simulink model "USV_Trajectory_Tracking_Control_Model"  (R2020b)
settings: Solver=ode4  StartTime=0.0  StopTime=400  FixedStep=0.01  RelTol=1e-3
libraries: simulink x15, sharedutil x6, aerolibutil x1
settings Model: Creator=cdsouza  LastModifiedBy=Admin
settings SolverCC: ZeroCrossAlgorithm=Adaptive
settings DataIOCC: ReturnWorkspaceOutputs=off
settings DebuggingCC: MaskedZcDiagnostic=none  IgnoredZcDiagnostic=none  ArithmeticOperatorsInVariantConditions=warning
settings SFSimCC: CustomCodeUndefinedFunction=UseInterfaceOnly

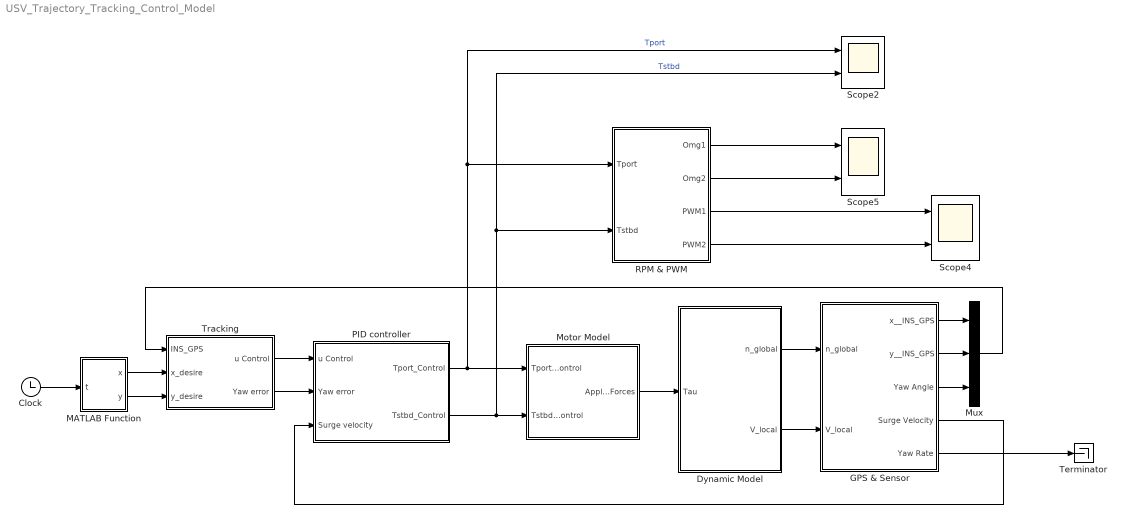
== system USV_Trajectory_Tracking_Control_Model ==
  Clock : Clock
  Dynamic Model : Subsystem
  GPS & Sensor : Subsystem
  MATLAB Function : MATLAB Function  TreatAsAtomicUnit=on
  Motor Model : Subsystem
  Mux : Mux  Inputs=3
  PID controller : Subsystem
  RPM & PWM : Subsystem
  Scope2 : Scope  NumInputPorts=2
  Scope4 : Scope  NumInputPorts=2
  Scope5 : Scope  NumInputPorts=2
  Terminator : Terminator
  Tracking : Subsystem
  wires:
  Tracking/1(u Control) -> PID controller/1(u Control)
  Tracking/2(Yaw error) -> PID controller/2(Yaw error)
  Dynamic Model/1(n_global) -> GPS & Sensor/1(n_global)
  Clock/1 -> MATLAB Function/1(t)
  MATLAB Function/1(x) -> Tracking/2(x_desire)
  MATLAB Function/2(y) -> Tracking/3(y_desire)
  PID controller/1(Tport_Control) -> Motor Model/1(Tport_Control), Scope2/1, RPM & PWM/1(Tport)  "Tport"
  PID controller/2(Tstbd_Control) -> Motor Model/2(Tstbd_Control), Scope2/2, RPM & PWM/2(Tstbd)  "Tstbd"
  GPS & Sensor/2(y__INS_GPS) -> Mux/2
  GPS & Sensor/1(x__INS_GPS) -> Mux/1
  GPS & Sensor/3(Yaw Angle) -> Mux/3
  Mux/1 -> Tracking/1(INS_GPS)
  GPS & Sensor/4(Surge Velocity) -> PID controller/3(Surge velocity)
  GPS & Sensor/5(Yaw Rate) -> Terminator/1
  RPM & PWM/3(PWM1) -> Scope4/1
  RPM & PWM/4(PWM2) -> Scope4/2
  Motor Model/1(Applied Forces) -> Dynamic Model/1(Tau)
  RPM & PWM/1(Omg1) -> Scope5/1
  RPM & PWM/2(Omg2) -> Scope5/2
  Dynamic Model/2(V_local) -> GPS & Sensor/2(V_local)

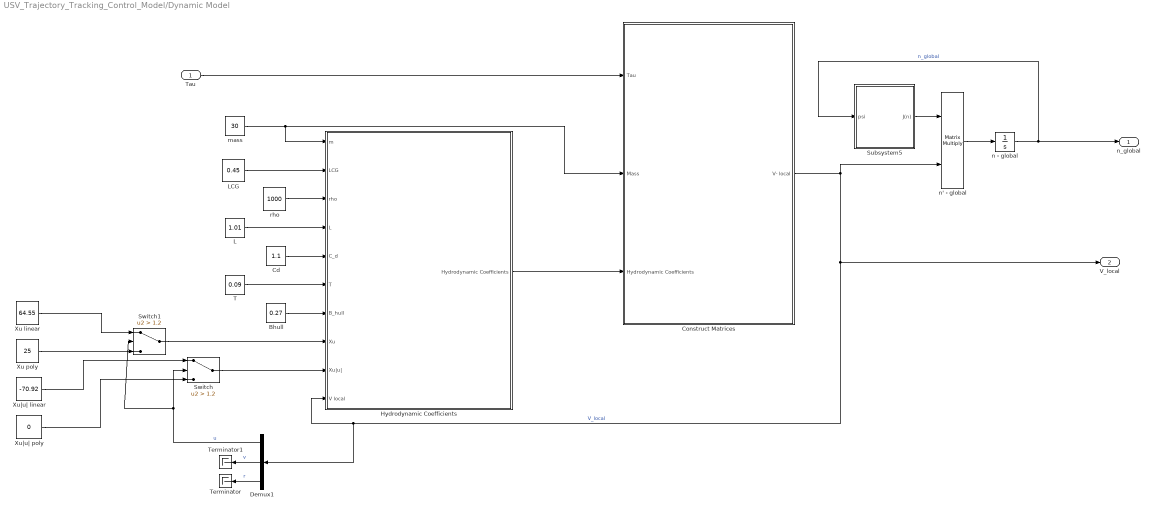
== system USV_Trajectory_Tracking_Control_Model/Dynamic Model ==
  Tau : Inport
  "Bhull " : Constant  Value=0.27
  Cd : Constant  Value=1.1
  Construct Matrices : Subsystem
  Demux1 : Demux  Outputs=3
  Hydrodynamic Coefficients : Subsystem
  L : Constant  Value=1.01
  LCG : Constant  Value=0.45
  Subsystem5 : Subsystem
  Switch : Switch  Criteria=u2 > Threshold  Threshold=1.2
  Switch1 : Switch  Criteria=u2 > Threshold  Threshold=1.2
  T : Constant  Value=0.09
  Terminator : Terminator
  Terminator1 : Terminator
  Xu linear : Constant  Value=64.55
  Xu poly : Constant  Value=25
  Xu|u| linear : Constant  Value=-70.92
  Xu|u| poly : Constant  Value=0
  mass : Constant  Value=30
  n - global : Integrator  InitialCondition=[0 0 0]
  n' - global : Product  Multiplication=Matrix(*)
  rho : Constant  Value=1000
  n_global : Outport  VectorParamsAs1DForOutWhenUnconnected=off
  V_local : Outport  Port=2  VectorParamsAs1DForOutWhenUnconnected=off
  wires:
  n - global/1 -> n_global/1, Subsystem5/1(psi)  "n_global"
  Cd/1 -> Hydrodynamic Coefficients/5(C_d)
  Construct Matrices/1(V- local) -> n' - global/2, Demux1/1, Hydrodynamic Coefficients/10(V local), V_local/1  "V_local"
  n' - global/1 -> n - global/1
  Subsystem5/1(J(n)) -> n' - global/1
  rho/1 -> Hydrodynamic Coefficients/3(rho)
  L/1 -> Hydrodynamic Coefficients/4(L)
  Tau/1 -> Construct Matrices/1(Tau)
  mass/1 -> Hydrodynamic Coefficients/1(m), Construct Matrices/2("Mass ")
  Hydrodynamic Coefficients/1("Hydrodynamic Coefficients ") -> Construct Matrices/3(Hydrodynamic Coefficients)
  T/1 -> Hydrodynamic Coefficients/6(T)
  "Bhull "/1 -> Hydrodynamic Coefficients/7(B_hull)
  Switch/1 -> Hydrodynamic Coefficients/9(Xu|u|)
  LCG/1 -> Hydrodynamic Coefficients/2(LCG)
  Demux1/1 -> Switch1/2, Switch/2  "u"
  Xu|u| poly/1 -> Switch/3
  Xu|u| linear/1 -> Switch/1
  Switch1/1 -> Hydrodynamic Coefficients/8(Xu)
  Xu poly/1 -> Switch1/3
  Xu linear/1 -> Switch1/1
  Demux1/3 -> Terminator/1  "r"
  Demux1/2 -> Terminator1/1  "v"

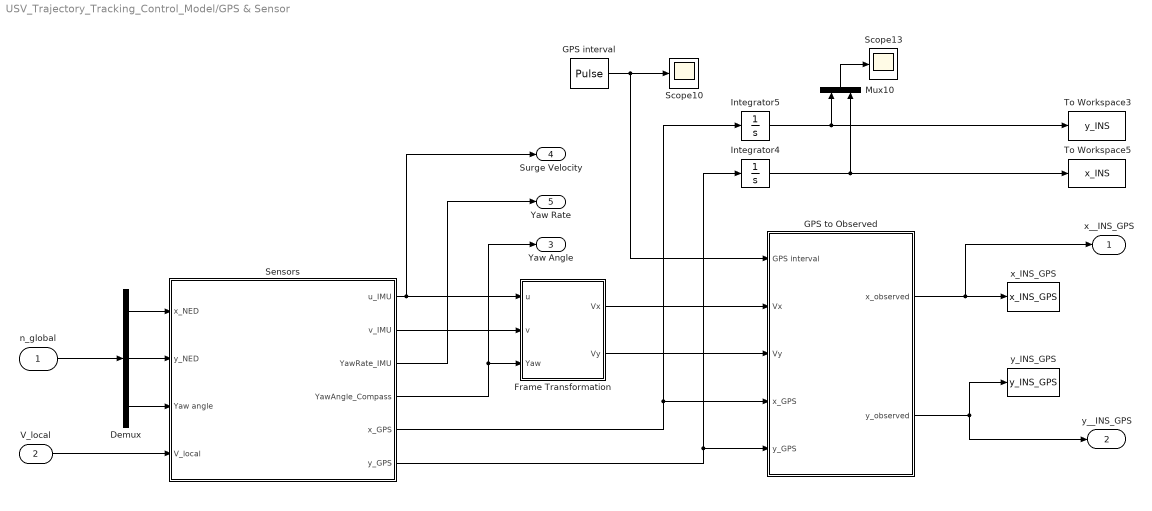
== system USV_Trajectory_Tracking_Control_Model/GPS & Sensor ==
  n_global : Inport
  V_local : Inport  Port=2
  Demux : Demux  Outputs=3
  Frame Transformation : Subsystem
  GPS interval : DiscretePulseGenerator  PulseType=Time based  Period=20  PulseWidth=5  PhaseDelay=0.2
  GPS to Observed : Subsystem
  Integrator4 : Integrator
  Integrator5 : Integrator
  Mux10 : Mux  Inputs=2
  Scope10 : Scope
  Scope13 : Scope
  Sensors : Subsystem
  To Workspace3 : ToWorkspace  VariableName=y_INS  SampleTime=-1
  To Workspace5 : ToWorkspace  VariableName=x_INS  SampleTime=-1
  x_INS_GPS : ToWorkspace  VariableName=x_INS_GPS  SampleTime=-1
  y_INS_GPS : ToWorkspace  VariableName=y_INS_GPS  SampleTime=-1
  x__INS_GPS : Outport  VectorParamsAs1DForOutWhenUnconnected=off
  y__INS_GPS : Outport  Port=2  VectorParamsAs1DForOutWhenUnconnected=off
  Yaw Angle : Outport  Port=3  VectorParamsAs1DForOutWhenUnconnected=off
  Surge Velocity : Outport  Port=4  VectorParamsAs1DForOutWhenUnconnected=off
  Yaw Rate : Outport  Port=5  VectorParamsAs1DForOutWhenUnconnected=off
  wires:
  GPS interval/1 -> GPS to Observed/1(GPS interval), Scope10/1
  Integrator5/1 -> To Workspace3/1, Mux10/1
  Sensors/1(u_IMU) -> Frame Transformation/1(u), Surge Velocity/1
  GPS to Observed/2(y_observed) -> y__INS_GPS/1, y_INS_GPS/1
  Mux10/1 -> Scope13/1
  GPS to Observed/1(x_observed) -> x__INS_GPS/1, x_INS_GPS/1
  Integrator4/1 -> To Workspace5/1, Mux10/2
  Sensors/2(v_IMU) -> Frame Transformation/2(v)
  Sensors/4(YawAngle_Compass) -> Yaw Angle/1, Frame Transformation/3(Yaw)
  Sensors/3(YawRate_IMU) -> Yaw Rate/1
  n_global/1 -> Demux/1
  Demux/3 -> Sensors/3(Yaw angle)
  Demux/1 -> Sensors/1(x_NED)
  Demux/2 -> Sensors/2(y_NED)
  V_local/1 -> Sensors/4(V_local)
  Sensors/6(y_GPS) -> Integrator4/1, GPS to Observed/5(y_GPS)
  Frame Transformation/2(Vy) -> GPS to Observed/3(Vy)
  Frame Transformation/1(Vx) -> GPS to Observed/2(Vx)
  Sensors/5(x_GPS) -> Integrator5/1, GPS to Observed/4(x_GPS)

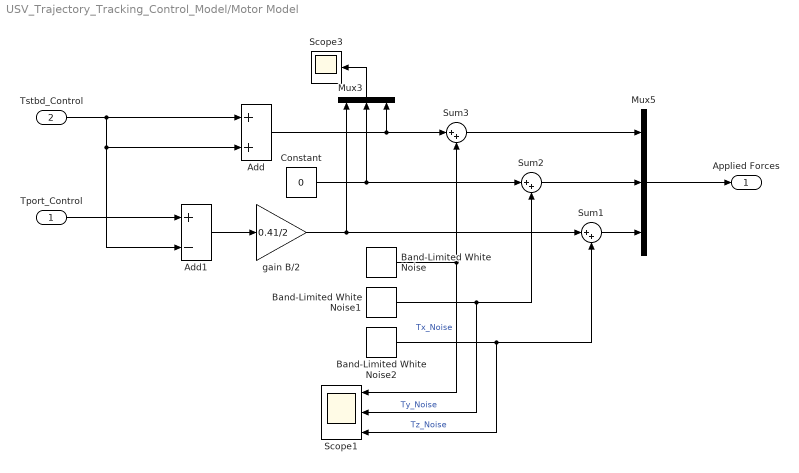
== system USV_Trajectory_Tracking_Control_Model/Motor Model ==
  Tport_Control : Inport
  Tstbd_Control : Inport  Port=2
  Add : Sum
  Add1 : Sum  Inputs=+-
  Band-Limited White Noise : simulink/Sources/Band-Limited White Noise  Cov=[0.05]  Ts=0.2  seed=[23341]
  Band-Limited White Noise1 : simulink/Sources/Band-Limited White Noise  Cov=[0.05]  Ts=0.2  seed=[23341]
  Band-Limited White Noise2 : simulink/Sources/Band-Limited White Noise  Cov=[0.05]  Ts=0.2  seed=[23341]
  Constant : Constant  Value=0
  Mux3 : Mux  Inputs=3
  Mux5 : Mux  Inputs=3
  Scope1 : Scope  NumInputPorts=3
  Scope3 : Scope
  Sum1 : Sum  Inputs=|++
  Sum2 : Sum  Inputs=|++
  Sum3 : Sum  Inputs=|++
  gain B/2 : Gain  Gain=0.41/2
  Applied Forces : Outport  VectorParamsAs1DForOutWhenUnconnected=off
  wires:
  Add1/1 -> gain B/2/1
  Tstbd_Control/1 -> Add1/2, Add/2, Add/1
  Add/1 -> Sum3/1, Mux3/3
  Tport_Control/1 -> Add1/1
  Constant/1 -> Mux3/2, Sum2/1
  Mux3/1 -> Scope3/1
  Band-Limited White Noise/1 -> Scope1/1, Sum3/2  "Tx_Noise"
  Mux5/1 -> Applied Forces/1
  Band-Limited White Noise2/1 -> Scope1/3, Sum1/2  "Tz_Noise"
  Sum3/1 -> Mux5/1
  Sum2/1 -> Mux5/2
  Sum1/1 -> Mux5/3
  gain B/2/1 -> Mux3/1, Sum1/1
  Band-Limited White Noise1/1 -> Scope1/2, Sum2/2  "Ty_Noise"

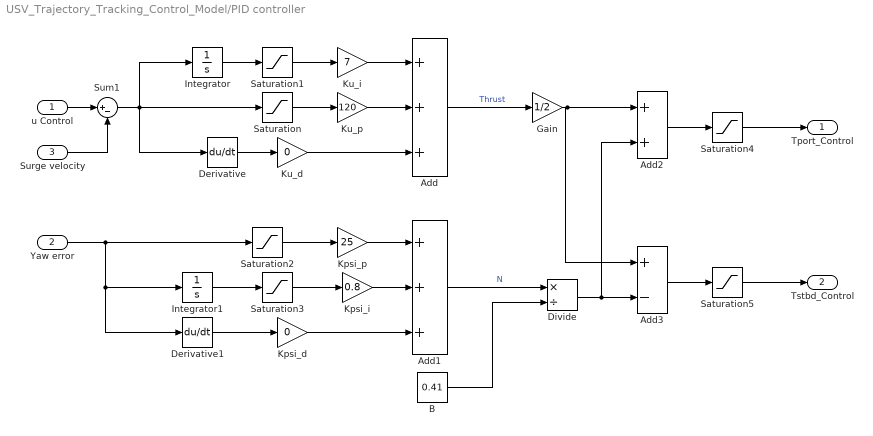
== system USV_Trajectory_Tracking_Control_Model/PID controller ==
  u Control : Inport
  Yaw error : Inport  Port=2
  Surge velocity : Inport  Port=3
  Add : Sum  Inputs=+++
  Add1 : Sum  Inputs=+++
  Add2 : Sum
  Add3 : Sum  Inputs=+-
  B : Constant  Value=0.41
  Derivative : Derivative
  Derivative1 : Derivative
  Divide : Product  Inputs=*/
  Gain : Gain  Gain=1/2
  Integrator : Integrator
  Integrator1 : Integrator
  Kpsi_d : Gain  Gain=0
  Kpsi_i : Gain  Gain=0.8
  Kpsi_p : Gain  Gain=25
  Ku_d : Gain  Gain=0
  Ku_i : Gain  Gain=7
  Ku_p : Gain  Gain=120
  Saturation : Saturate  UpperLimit=3  LowerLimit=0
  Saturation1 : Saturate  UpperLimit=10  LowerLimit=-10
  Saturation2 : Saturate  UpperLimit=0.8
  Saturation3 : Saturate  UpperLimit=10  LowerLimit=-10
  Saturation4 : Saturate  UpperLimit=25  LowerLimit=0
  Saturation5 : Saturate  UpperLimit=25  LowerLimit=0
  Sum1 : Sum  Inputs=|+-
  Tport_Control : Outport  VectorParamsAs1DForOutWhenUnconnected=off
  Tstbd_Control : Outport  Port=2  VectorParamsAs1DForOutWhenUnconnected=off
  wires:
  Integrator1/1 -> Saturation3/1
  Yaw error/1 -> Saturation2/1, Derivative1/1, Integrator1/1
  Surge velocity/1 -> Sum1/2
  u Control/1 -> Sum1/1
  Sum1/1 -> Derivative/1, Saturation/1, Integrator/1
  Integrator/1 -> Saturation1/1
  Saturation1/1 -> Ku_i/1
  Saturation/1 -> Ku_p/1
  Ku_p/1 -> Add/2
  Ku_i/1 -> Add/1
  Saturation2/1 -> Kpsi_p/1
  Saturation3/1 -> Kpsi_i/1
  Kpsi_p/1 -> Add1/1
  Kpsi_i/1 -> Add1/2
  Add/1 -> Gain/1  "Thrust"
  Add1/1 -> Divide/1  "N"
  B/1 -> Divide/2
  Gain/1 -> Add3/1, Add2/1
  Divide/1 -> Add3/2, Add2/2
  Add2/1 -> Saturation4/1
  Add3/1 -> Saturation5/1
  Derivative/1 -> Ku_d/1
  Ku_d/1 -> Add/3
  Derivative1/1 -> Kpsi_d/1
  Kpsi_d/1 -> Add1/3
  Saturation4/1 -> Tport_Control/1
  Saturation5/1 -> Tstbd_Control/1

== system USV_Trajectory_Tracking_Control_Model/RPM & PWM ==
  Tport : Inport
  Tstbd : Inport  Port=2
  Add : Sum
  Clock : Clock
  Constant : Constant  Value=3977
  Demux1 : Demux  Outputs=2
  Demux2 : Demux  Outputs=2
  Gain : Gain  Gain=1/(2e-6)
  Gain1 : Gain  Gain=1/79540
  Mux1 : Mux  Inputs=2
  PWM sim1 : MATLAB Function  TreatAsAtomicUnit=on
  PWM sim2 : MATLAB Function  TreatAsAtomicUnit=on
  Signed Square Root : Sqrt  Operator=signedSqrt  SaturateOnIntegerOverflow=on
  Omg1 : Outport
  Omg2 : Outport  Port=2
  PWM1 : Outport  Port=3
  PWM2 : Outport  Port=4
  wires:
  Mux1/1 -> Gain/1
  Tstbd/1 -> Mux1/2  "Tstbd"
  Tport/1 -> Mux1/1  "Tport"
  Gain/1 -> Signed Square Root/1
  Signed Square Root/1 -> Add/1, Demux2/1
  Add/1 -> Gain1/1
  Gain1/1 -> Demux1/1
  Demux1/1 -> PWM sim1/2(sig)
  Demux1/2 -> PWM sim2/2(sig)
  Clock/1 -> PWM sim2/1(rtime), PWM sim1/1(rtime)
  PWM sim1/1(pwm_wave) -> PWM1/1  "pwm"
  PWM sim2/1(pwm_wave) -> PWM2/1  "pwm"
  Constant/1 -> Add/2
  Demux2/1 -> Omg1/1
  Demux2/2 -> Omg2/1

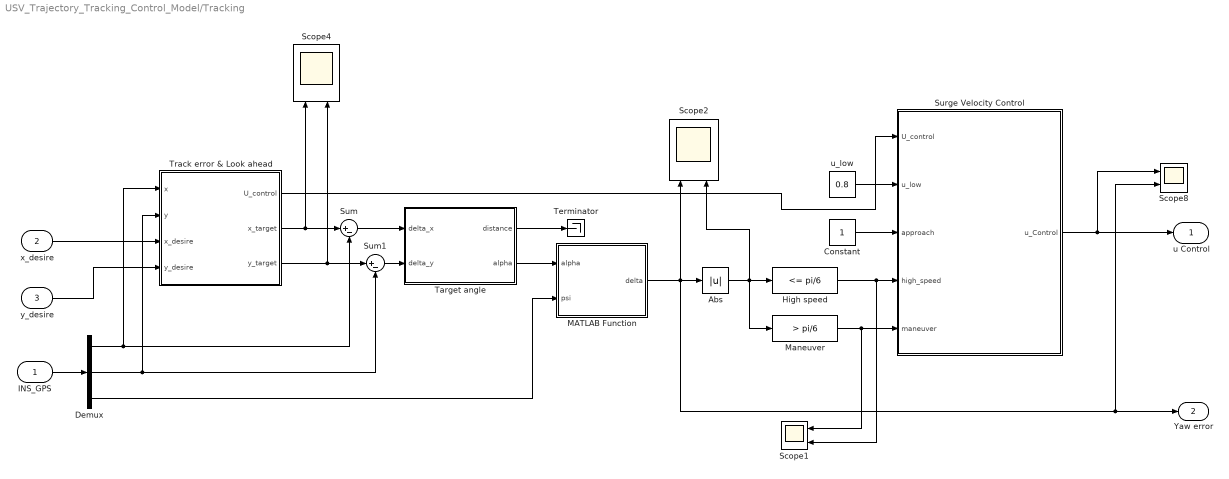
== system USV_Trajectory_Tracking_Control_Model/Tracking ==
  INS_GPS : Inport
  x_desire : Inport  Port=2
  y_desire : Inport  Port=3
  Abs : Abs
  Constant : Constant
  Demux : Demux  Outputs=3
  High speed : simulink/Logic and Bit Operations/Compare To Constant  relop=<=  const=pi/6  OutDataTypeStr=boolean
  MATLAB Function : MATLAB Function  TreatAsAtomicUnit=on
  Maneuver : simulink/Logic and Bit Operations/Compare To Constant  relop=>  const=pi/6  OutDataTypeStr=boolean
  Scope{1..2,4,8} (4 alike) : Scope  NumInputPorts=2
  Sum : Sum  Inputs=|+-
  Sum1 : Sum  Inputs=|+-
  Surge Velocity Control : MATLAB Function  TreatAsAtomicUnit=on
  Target angle : MATLAB Function  TreatAsAtomicUnit=on
  Terminator : Terminator
  Track error & Look ahead : Subsystem
  u_low : Constant  Value=0.8
  u Control : Outport  VectorParamsAs1DForOutWhenUnconnected=off
  Yaw error : Outport  Port=2  VectorParamsAs1DForOutWhenUnconnected=off
  wires:
  Target angle/2(alpha) -> MATLAB Function/1(alpha)
  Maneuver/1 -> Scope1/1, Surge Velocity Control/5(maneuver)
  Sum/1 -> Target angle/1(delta_x)
  u_low/1 -> Surge Velocity Control/2(u_low)
  Abs/1 -> High speed/1, Maneuver/1, Scope2/2
  Sum1/1 -> Target angle/2(delta_y)
  Demux/2 -> Sum1/2, Track error & Look ahead/2(y)
  MATLAB Function/1(delta) -> Scope2/1, Abs/1, Scope8/2, Yaw error/1
  High speed/1 -> Scope1/2, Surge Velocity Control/4(high_speed)
  Demux/1 -> Sum/2, Track error & Look ahead/1(x)
  Surge Velocity Control/1(u_Control) -> Scope8/1, u Control/1
  Demux/3 -> MATLAB Function/2(psi)
  Track error & Look ahead/2(x_target) -> Sum/1, Scope4/1
  Track error & Look ahead/3(y_target) -> Scope4/2, Sum1/1
  Target angle/1(distance) -> Terminator/1
  Track error & Look ahead/1(U_control) -> Surge Velocity Control/1(U_control)
  Constant/1 -> Surge Velocity Control/3(approach)
  INS_GPS/1 -> Demux/1
  x_desire/1 -> Track error & Look ahead/3(x_desire)
  y_desire/1 -> Track error & Look ahead/4(y_desire)

== system USV_Trajectory_Tracking_Control_Model/Dynamic Model/Construct Matrices ==
  note: v' local
  Tau : Inport
  "Mass " : Inport  Port=2
  Hydrodynamic Coefficients : Inport  Port=3
  I : Constant  Value=4.1
  Integrator : Integrator
  M : Subsystem
  M^-1 : aerolibutil/Invert  3x3 Matrix
  M^-1(T-C(v)-D(v)) : Product  Multiplication=Matrix(*)
  T-C(v)-D(v) : Subsystem
  XG : Constant  Value=0
  YG : Constant  Value=0
  V- local : Outport  VectorParamsAs1DForOutWhenUnconnected=off
  wires:
  M/1(M) -> M^-1/1  "M"
  Integrator/1 -> V- local/1, T-C(v)-D(v)/4(V_Local)  "V_Local"
  M^-1(T-C(v)-D(v))/1 -> Integrator/1
  I/1 -> M/4(I_z)
  M^-1/1 -> M^-1(T-C(v)-D(v))/1
  Hydrodynamic Coefficients/1 -> T-C(v)-D(v)/5(HydrodynamicCoefficients), M/5(Hydrodynamic coefficients)  "HydrodynamicCoefficients"
  YG/1 -> T-C(v)-D(v)/3(Y_G), M/3(Y_G)
  "Mass "/1 -> T-C(v)-D(v)/1(m), M/1(m)
  XG/1 -> T-C(v)-D(v)/2(X_G), M/2(X_G)
  T-C(v)-D(v)/1(Out1) -> M^-1(T-C(v)-D(v))/2
  Tau/1 -> T-C(v)-D(v)/6(Tau)

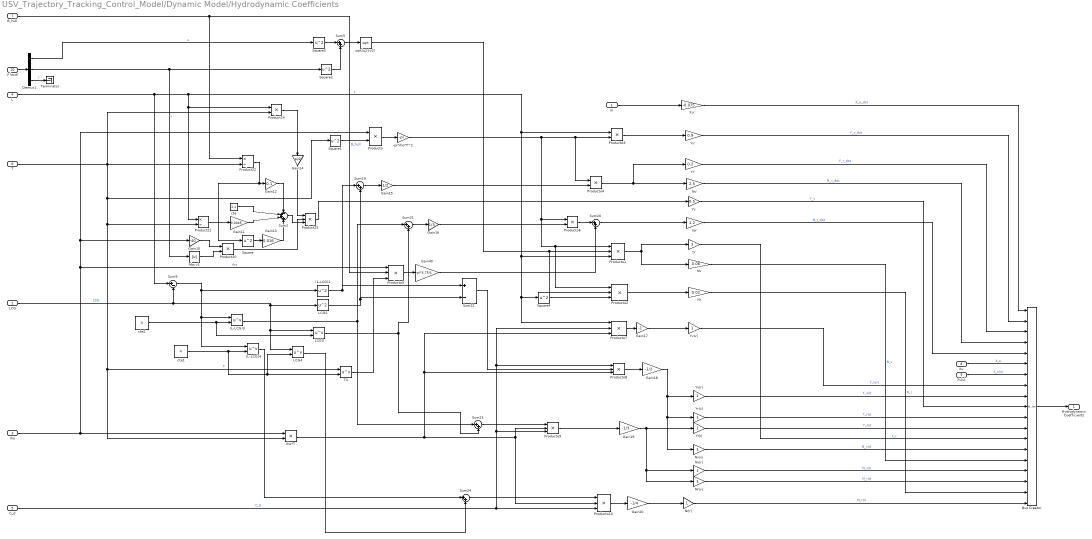
== system USV_Trajectory_Tracking_Control_Model/Dynamic Model/Hydrodynamic Coefficients ==
  m : Inport
  LCG : Inport  Port=2
  rho : Inport  Port=3
  L : Inport  Port=4
  C_d : Inport  Port=5
  T : Inport  Port=6
  B_hull : Inport  Port=7
  Xu : Inport  Port=8
  Xu|u| : Inport  Port=9
  V local : Inport  Port=10
  (L-LCG)2 : Math  Operator=square  SignedPower=on  SaturateOnIntegerOverflow=on
  (L-LCG)3 : Math  Operator=pow  SignedPower=on  SaturateOnIntegerOverflow=on
  (L-LCG)4 : Math  Operator=pow  SignedPower=on  SaturateOnIntegerOverflow=on
  -pi*rho*T^2 : Gain  Gain=-pi
  Abs v1 : Abs
  Bus Creator : BusCreator  Inputs=19
  Demux1 : Demux  Outputs=3
  Gain10 : Gain  Gain=-40
  Gain11 : Gain  Gain=0.0045
  Gain12 : Gain  Gain=0.1
  Gain13 : Gain  Gain=0.016
  Gain14 : Gain  Gain=pi/2
  Gain15 : Gain  Gain=1/2
  Gain16 : Gain  Gain=1/3
  Gain17 : Gain  Gain=-1
  Gain18 : Gain  Gain=-1/2
  Gain19 : Gain  Gain=-1/3
  Gain20 : Gain  Gain=-1/4
  Gain40 : Gain  Gain=-pi*4.75/4
  LCG2 : Math  Operator=square  SignedPower=on  SaturateOnIntegerOverflow=on
  LCG3 : Math  Operator=pow  SignedPower=on  SaturateOnIntegerOverflow=on
  LCG4 : Math  Operator=pow  SignedPower=on  SaturateOnIntegerOverflow=on
  Nr : Gain  Gain=0.02
  Nr' : Gain  Gain=1.2
  Nr|r| : Gain
  Nr|v| : Gain
  Nv : Gain  Gain=0.06
  Nv' : Gain  Gain=2.5
  Nv|r| : Gain
  Nv|v| : Gain
  Product20 : Product
  Product21 : Product  Inputs=*/
  Product22 : Product  Inputs=*/
  Product23 : Product  Inputs=3
  Product24 : Product
  Producto{,3..4,6} (4 alike) : Product
  Producto{1..2,5,7..10} (7 alike) : Product  Inputs=3
  Square{,1..4} (5 alike) : Math  Operator=square  SignedPower=on  SaturateOnIntegerOverflow=on
  Sum{5,19..21,23..24} (6 alike) : Sum  Inputs=|++
  Sum2 : Sum  Inputs=-+++
  Sum22 : Sum  Inputs=|+-
  Sum9 : Sum  Inputs=|+-
  T4 : Math  Operator=pow  SignedPower=on  SaturateOnIntegerOverflow=on
  Terminator : Terminator
  Xu' : Gain  Gain=-0.075
  Yr : Gain  Gain=3
  Yr' : Gain  Gain=0.2
  Yr|r| : Gain
  Yr|v| : Gain
  Yv : Gain  Gain=0.5
  Yv' : Gain  Gain=0.9
  Yv|r| : Gain
  Yv|v| : Gain
  cte : Constant  Value=1.1
  cte1 : Constant  Value=4
  cte2 : Constant  Value=3
  rho*T : Product
  sqrt(u2+v2) : Sqrt  SaturateOnIntegerOverflow=on
  "Hydrodynamic Coefficients " : Outport  VectorParamsAs1DForOutWhenUnconnected=off
  wires:
  m/1 -> Xu'/1
  Nv'/1 -> Bus Creator/4  "N_v_dot"
  Xu'/1 -> Bus Creator/1  "X_u_dot"
  Square/1 -> Gain13/1
  Gain14/1 -> Product23/1
  Product24/1 -> Gain14/1
  Sum9/1 -> (L-LCG)3/1, (L-LCG)4/1, (L-LCG)2/1
  Square4/1 -> Producto2/3
  sqrt(u2+v2)/1 -> Producto2/2, Producto1/2
  Product20/1 -> Product23/2
  Gain13/1 -> Sum2/4
  B_hull/1 -> Producto5/2, Product22/1  "B_hull"
  Square2/1 -> Sum5/2
  Sum20/1 -> Nr'/1
  Gain12/1 -> Sum2/1
  Sum21/1 -> Gain16/1
  LCG4/1 -> Sum24/2
  Sum24/1 -> Producto10/1
  (L-LCG)4/1 -> Sum24/1
  Sum2/1 -> Product23/3
  Producto10/1 -> Gain20/1
  (L-LCG)3/1 -> Sum21/1, Sum23/1
  Producto6/1 -> Sum20/1
  Gain19/1 -> Yr|r|/1, Nr|v|/1, Nv|r|/1
  Gain16/1 -> Producto6/2
  Sum22/1 -> Producto8/2
  Producto3/1 -> Yv'/1
  Gain10/1 -> Product20/1
  cte1/1 -> LCG4/2, T4/2, (L-LCG)4/2
  cte2/1 -> (L-LCG)3/2, LCG3/2
  Product23/1 -> Yv/1
  cte/1 -> Sum2/2
  Producto8/1 -> Gain18/1
  Sum23/1 -> Producto9/1
  Gain20/1 -> Nr|r|/1
  Gain18/1 -> Nv|v|/1, Yr|v|/1, Yv|r|/1
  Yr'/1 -> Bus Creator/3  "Y_r_dot"
  Producto7/1 -> Gain17/1
  Producto9/1 -> Gain19/1
  Gain11/1 -> Sum2/3
  Square1/1 -> Producto/2
  Producto2/1 -> Nr/1
  LCG3/1 -> Sum21/2, Sum23/2
  T4/1 -> Producto5/3
  Gain40/1 -> Sum20/2
  Producto4/1 -> Yr'/1, Nv'/1
  Sum19/1 -> Gain15/1
  Square3/1 -> Sum5/1
  Sum5/1 -> sqrt(u2+v2)/1
  rho/1 -> Producto/1, Gain10/1, Producto5/1, rho*T/1  "rho"
  Abs v1/1 -> Product20/2
  Product21/1 -> Gain11/1
  Gain17/1 -> Yv|v|/1
  (L-LCG)2/1 -> Sum19/1, Sum22/1
  Producto1/1 -> Nv/1, Yr/1
  Product22/1 -> Square/1, Gain12/1
  LCG2/1 -> Sum19/2, Sum22/2
  LCG/1 -> Sum9/2, LCG2/1, LCG3/1, LCG4/1  "LCG"
  Producto/1 -> -pi*rho*T^2/1
  -pi*rho*T^2/1 -> Producto4/1, Producto3/2, Producto2/1, Producto1/1, Producto6/1
  Producto5/1 -> Gain40/1
  Gain15/1 -> Producto4/2
  rho*T/1 -> Producto9/2, Producto10/2, Producto7/3, Producto8/3
  T/1 -> Product21/2, rho*T/2, T4/1, Square1/1, Product22/2, Product24/2  "T"
  L/1 -> Producto7/1, Square4/1, Producto1/3, Producto3/1, Product21/1, Product24/1, Sum9/1  "L"
  C_d/1 -> Producto7/2, Producto8/1, Producto9/3, Producto10/3  "C_d"
  Nv/1 -> Bus Creator/15  "N_v"
  Yv|v|/1 -> Bus Creator/8  "Y_v|v|"
  Yr|r|/1 -> Bus Creator/12  "Y_r|r|"
  Yv/1 -> Bus Creator/10  "Y_v"
  Nv|v|/1 -> Bus Creator/14  "N_v|v|"
  Yr|v|/1 -> Bus Creator/11  "Y_r|v|"
  Nv|r|/1 -> Bus Creator/16  "N_v|r|"
  Yr/1 -> Bus Creator/13  "Y_r"
  Nr|r|/1 -> Bus Creator/19  "N_r|r|"
  Nr/1 -> Bus Creator/18  "N_r"
  Xu|u|/1 -> Bus Creator/7  "X_u|u|"
  Yv|r|/1 -> Bus Creator/9  "Y_v|r|"
  Nr|v|/1 -> Bus Creator/17  "N_r|v|"
  Xu/1 -> Bus Creator/6  "X_u"
  Bus Creator/1 -> "Hydrodynamic Coefficients "/1
  Nr'/1 -> Bus Creator/5  "N_r_dot"
  Yv'/1 -> Bus Creator/2  "Y_v_dot"
  Demux1/1 -> Square3/1  "u"
  V local/1 -> Demux1/1
  Demux1/2 -> Abs v1/1, Square2/1  "v"
  Demux1/3 -> Terminator/1  "r"

== system USV_Trajectory_Tracking_Control_Model/Dynamic Model/Subsystem5 ==
  psi : Inport
  " J(n)" : sharedutil/Create 3x3 Matrix  aMode=aMode
      settings: SourceProductBaseCode=AE,PW,MT,UV,VE,VP
  Constant1 : Constant
  Constant2 : Constant  Value=0
  Gain9 : Gain  Gain=-1
  Selector : Selector  InputPortWidth=3  IndexOptions=Index vector (dialog)  Indices=3  OutputSizes=1
  Trigonometric Function : Trigonometry
  Trigonometric Function1 : Trigonometry  Operator=cos
  J(n) : Outport  VectorParamsAs1DForOutWhenUnconnected=off
  wires:
  Gain9/1 -> " J(n)"/2
  Trigonometric Function1/1 -> " J(n)"/5, " J(n)"/1
  Trigonometric Function/1 -> " J(n)"/4, Gain9/1
  Constant1/1 -> " J(n)"/9
  psi/1 -> Selector/1
  " J(n)"/1 -> J(n)/1
  Constant2/1 -> " J(n)"/8, " J(n)"/7, " J(n)"/6, " J(n)"/3
  Selector/1 -> Trigonometric Function1/1, Trigonometric Function/1

== system USV_Trajectory_Tracking_Control_Model/GPS & Sensor/Frame Transformation ==
  u : Inport
  v : Inport  Port=2
  Yaw : Inport  Port=3
  MATLAB Function : MATLAB Function  TreatAsAtomicUnit=on
  Vx : Outport  VectorParamsAs1DForOutWhenUnconnected=off
  Vy : Outport  Port=2  VectorParamsAs1DForOutWhenUnconnected=off
  wires:
  Yaw/1 -> MATLAB Function/3(Yaw)
  MATLAB Function/2(Vy_0) -> Vy/1
  u/1 -> MATLAB Function/1(u)
  MATLAB Function/1(Vx_0) -> Vx/1
  v/1 -> MATLAB Function/2(v)

== system USV_Trajectory_Tracking_Control_Model/GPS & Sensor/GPS to Observed ==
  GPS interval : Inport
  Vx : Inport  Port=2
  Vy : Inport  Port=3
  x_GPS : Inport  Port=4
  y_GPS : Inport  Port=5
  Mux6 : Mux  Inputs=2
  Scope8 : Scope
  x_inferred : Integrator  ExternalReset=rising  InitialConditionSource=external
  y_inferred : Integrator  ExternalReset=rising  InitialConditionSource=external
  x_observed : Outport  VectorParamsAs1DForOutWhenUnconnected=off
  y_observed : Outport  Port=2  VectorParamsAs1DForOutWhenUnconnected=off
  wires:
  y_inferred/1 -> y_observed/1, Mux6/1
  Vy/1 -> y_inferred/1
  GPS interval/1 -> y_inferred/2, x_inferred/2
  Vx/1 -> x_inferred/1
  x_inferred/1 -> x_observed/1, Mux6/2
  Mux6/1 -> Scope8/1
  y_GPS/1 -> y_inferred/3
  x_GPS/1 -> x_inferred/3

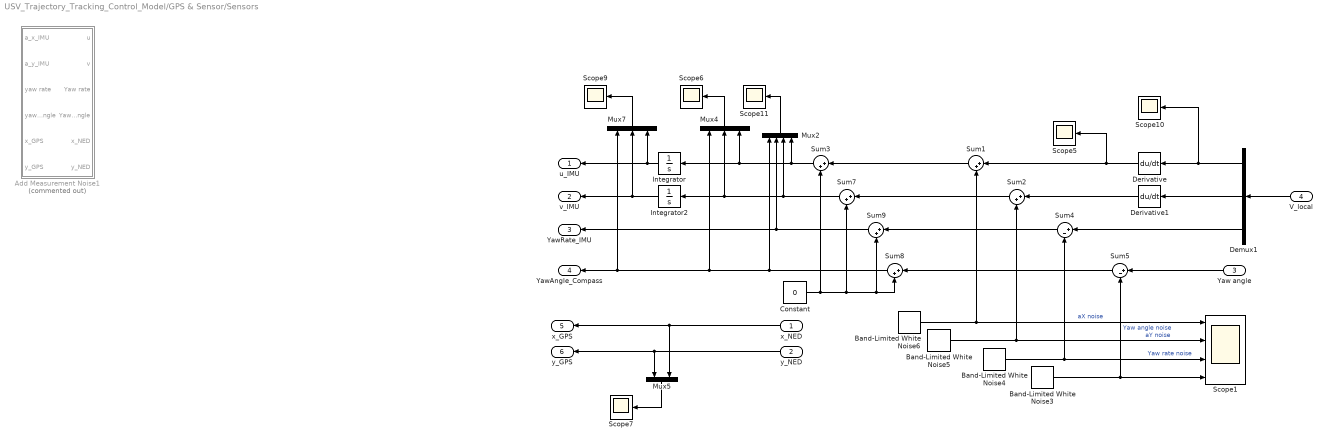
== system USV_Trajectory_Tracking_Control_Model/GPS & Sensor/Sensors ==
  x_NED : Inport
  y_NED : Inport  Port=2
  Yaw angle : Inport  Port=3
  V_local : Inport  Port=4
  Add Measurement Noise1 : Subsystem  Commented=on
  Band-Limited White Noise3 : simulink/Sources/Band-Limited White Noise  Cov=[0.0001]  Ts=0.1  seed=[23341]
  Band-Limited White Noise4 : simulink/Sources/Band-Limited White Noise  Cov=[0.00000001]  Ts=0.1  seed=[23341]
  Band-Limited White Noise5 : simulink/Sources/Band-Limited White Noise  Cov=[0.00000005]  Ts=0.1  seed=[23341]
  Band-Limited White Noise6 : simulink/Sources/Band-Limited White Noise  Cov=[0.000005]  Ts=0.1  seed=[23341]
  Constant : Constant  Value=0
  Demux1 : Demux  Outputs=3
  Derivative : Derivative
  Derivative1 : Derivative
  Integrator : Integrator
  Integrator2 : Integrator
  Mux2 : Mux
  Mux4 : Mux  Inputs=3
  Mux5 : Mux  Inputs=2
  Mux7 : Mux  Inputs=3
  Scope1 : Scope  NumInputPorts=4
  Scope{5..7,9..11} (6 alike) : Scope
  Sum{1..3,7..9} (6 alike) : Sum  Inputs=|++
  Sum4 : Sum  Inputs=|+-
  Sum5 : Sum  Inputs=|+-
  u_IMU : Outport  VectorParamsAs1DForOutWhenUnconnected=off
  v_IMU : Outport  Port=2  VectorParamsAs1DForOutWhenUnconnected=off
  YawRate_IMU : Outport  Port=3  VectorParamsAs1DForOutWhenUnconnected=off
  YawAngle_Compass : Outport  Port=4  VectorParamsAs1DForOutWhenUnconnected=off
  x_GPS : Outport  Port=5  VectorParamsAs1DForOutWhenUnconnected=off
  y_GPS : Outport  Port=6  VectorParamsAs1DForOutWhenUnconnected=off
  wires:
  Mux7/1 -> Scope9/1
  Sum3/1 -> Mux4/3, Integrator/1, Mux2/4
  Integrator/1 -> Mux7/3, u_IMU/1
  x_NED/1 -> Mux5/2, x_GPS/1
  Sum7/1 -> Mux4/2, Integrator2/1, Mux2/3
  Mux4/1 -> Scope6/1
  Integrator2/1 -> Mux7/2, v_IMU/1
  Mux5/1 -> Scope7/1
  Sum8/1 -> Mux2/1, Mux4/1, Mux7/1, YawAngle_Compass/1
  y_NED/1 -> y_GPS/1, Mux5/1
  Sum9/1 -> Mux2/2, YawRate_IMU/1
  V_local/1 -> Demux1/1
  Sum4/1 -> Sum9/1
  Sum5/1 -> Sum8/1
  Band-Limited White Noise6/1 -> Sum1/2, Scope1/1  "aX noise"
  Sum2/1 -> Sum7/1
  Mux2/1 -> Scope11/1
  Sum1/1 -> Sum3/1
  Band-Limited White Noise3/1 -> Sum5/2, Scope1/4  "Yaw angle noise"
  Demux1/3 -> Sum4/1
  Constant/1 -> Sum8/2, Sum9/2, Sum7/2, Sum3/2
  Derivative1/1 -> Sum2/1
  Demux1/1 -> Scope10/1, Derivative/1
  Yaw angle/1 -> Sum5/1
  Derivative/1 -> Scope5/1, Sum1/1
  Band-Limited White Noise5/1 -> Scope1/2, Sum2/2  "aY noise"
  Demux1/2 -> Derivative1/1
  Band-Limited White Noise4/1 -> Scope1/3, Sum4/2  "Yaw rate noise"

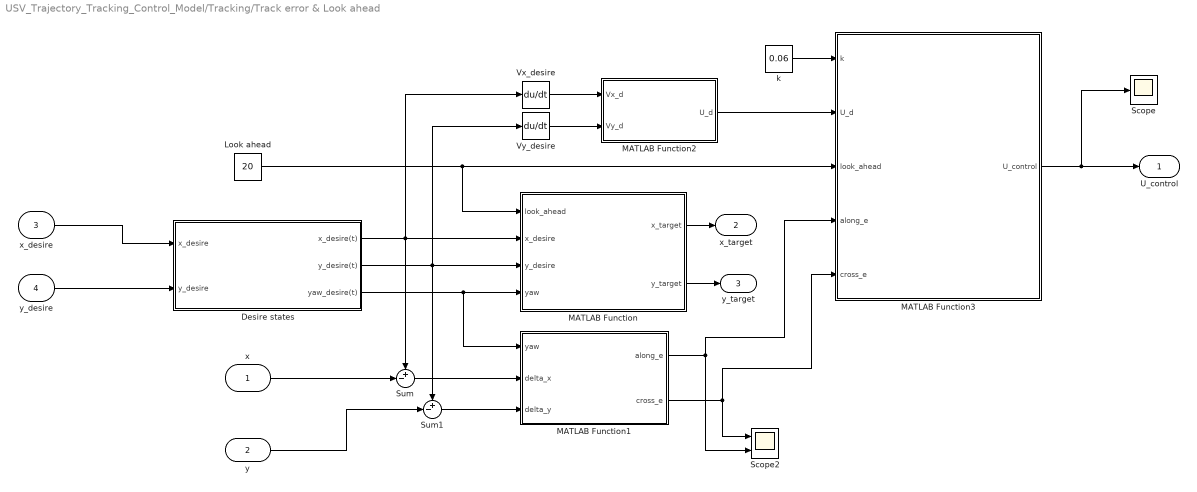
== system USV_Trajectory_Tracking_Control_Model/Tracking/Track error & Look ahead ==
  x : Inport
  y : Inport  Port=2
  x_desire : Inport  Port=3
  y_desire : Inport  Port=4
  Desire states : Subsystem
  Look ahead : Constant  Value=20
  MATLAB Function : MATLAB Function  TreatAsAtomicUnit=on
  MATLAB Function1 : MATLAB Function  TreatAsAtomicUnit=on
  MATLAB Function2 : MATLAB Function  TreatAsAtomicUnit=on
  MATLAB Function3 : MATLAB Function  TreatAsAtomicUnit=on
  Scope : Scope
  Scope2 : Scope  NumInputPorts=2
  Sum : Sum  Inputs=+-|
  Sum1 : Sum  Inputs=+-|
  Vx_desire : Derivative
  Vy_desire : Derivative
  k : Constant  Value=0.06
  U_control : Outport  VectorParamsAs1DForOutWhenUnconnected=off
  x_target : Outport  Port=2  VectorParamsAs1DForOutWhenUnconnected=off
  y_target : Outport  Port=3  VectorParamsAs1DForOutWhenUnconnected=off
  wires:
  Desire states/3(yaw_desire(t)) -> MATLAB Function1/1(yaw), MATLAB Function/4(yaw)
  Desire states/1(x_desire(t)) -> Vx_desire/1, MATLAB Function/2(x_desire), Sum/1
  Desire states/2(y_desire(t)) -> Sum1/1, MATLAB Function/3(y_desire), Vy_desire/1
  Look ahead/1 -> MATLAB Function/1(look_ahead), MATLAB Function3/3(look_ahead)
  MATLAB Function/1(x_target) -> x_target/1
  MATLAB Function/2(y_target) -> y_target/1
  x/1 -> Sum/2
  y/1 -> Sum1/2
  Sum1/1 -> MATLAB Function1/3(delta_y)
  Sum/1 -> MATLAB Function1/2(delta_x)
  Vx_desire/1 -> MATLAB Function2/1(Vx_d)
  Vy_desire/1 -> MATLAB Function2/2(Vy_d)
  MATLAB Function2/1(U_d) -> MATLAB Function3/2(U_d)
  MATLAB Function1/1(along_e) -> Scope2/2, MATLAB Function3/4(along_e)
  MATLAB Function1/2(cross_e) -> Scope2/1, MATLAB Function3/5(cross_e)
  k/1 -> MATLAB Function3/1(k)
  MATLAB Function3/1(U_control) -> Scope/1, U_control/1
  x_desire/1 -> Desire states/1(x_desire)
  y_desire/1 -> Desire states/2(y_desire)

== system USV_Trajectory_Tracking_Control_Model/Dynamic Model/Construct Matrices/M ==
  m : Inport
  X_G : Inport  Port=2
  Y_G : Inport  Port=3
  I_z : Inport  Port=4
  Hydrodynamic coefficients : Inport  Port=5
  Bus Selector : BusSelector  OutputSignals=X_u_dot,Y_r_dot,N_v_dot,Y_v_dot,N_r_dot
  Constant3 : Constant  Value=0
  Gain8 : Gain  Gain=-1
  Matrix M : sharedutil/Create 3x3 Matrix  aMode=aMode
      settings: SourceProductBaseCode=AE,PW,MT,UV,VE,VP
  Product17 : Product
  Product18 : Product
  Sum14 : Sum  Inputs=|+-
  Sum15 : Sum  Inputs=+-
  Sum16 : Sum  Inputs=+-
  Sum17 : Sum  Inputs=+-
  Sum18 : Sum  Inputs=|+-
  M : Outport  VectorParamsAs1DForOutWhenUnconnected=off
  wires:
  Gain8/1 -> Matrix M/7, Matrix M/3
  Product17/1 -> Gain8/1
  Product18/1 -> Sum17/1, Sum16/1
  Sum18/1 -> Matrix M/9
  Constant3/1 -> Matrix M/4, Matrix M/2
  I_z/1 -> Sum18/1  "I_z"
  Sum15/1 -> Matrix M/5
  m/1 -> Sum14/1, Product17/1, Sum15/1, Product18/1  "m"
  Bus Selector/3 -> Sum17/2  "<N_v_dot>"
  Sum14/1 -> Matrix M/1
  Sum16/1 -> Matrix M/6
  Matrix M/1 -> M/1
  Sum17/1 -> Matrix M/8
  X_G/1 -> Product18/2  "X_G"
  Y_G/1 -> Product17/2  "Y_G"
  Bus Selector/1 -> Sum14/2  "<X_u_dot>"
  Hydrodynamic coefficients/1 -> Bus Selector/1
  Bus Selector/2 -> Sum16/2  "<Y_r_dot>"
  Bus Selector/4 -> Sum15/2  "<Y_v_dot>"
  Bus Selector/5 -> Sum18/2  "<N_r_dot>"

== system USV_Trajectory_Tracking_Control_Model/Dynamic Model/Construct Matrices/T-C(v)-D(v) ==
  m : Inport
  X_G : Inport  Port=2
  Y_G : Inport  Port=3
  V_Local : Inport  Port=4
  HydrodynamicCoefficients : Inport  Port=5
  Tau : Inport  Port=6
  C : Subsystem
  C(v)v : Product  Multiplication=Matrix(*)
  D : Subsystem
  D(v)v : Product  Multiplication=Matrix(*)
  T - C(v)v - D(v)v : Sum  Inputs=+--
  Out1 : Outport  VectorParamsAs1DForOutWhenUnconnected=off
  wires:
  V_Local/1 -> D(v)v/2, C(v)v/2, D/2(V - local), C/5(V local)
  T - C(v)v - D(v)v/1 -> Out1/1
  D(v)v/1 -> T - C(v)v - D(v)v/3
  C(v)v/1 -> T - C(v)v - D(v)v/2
  C/1(C(v)) -> C(v)v/1  "C(v)"
  D/1(D(v)) -> D(v)v/1  "D(v)"
  HydrodynamicCoefficients/1 -> C/4(Hydrodynamic coefficients), D/1(Hydrodynamic Coefficients)
  Y_G/1 -> C/3(Y_G)
  X_G/1 -> C/2(X_G)
  m/1 -> C/1(m)
  Tau/1 -> T - C(v)v - D(v)v/1

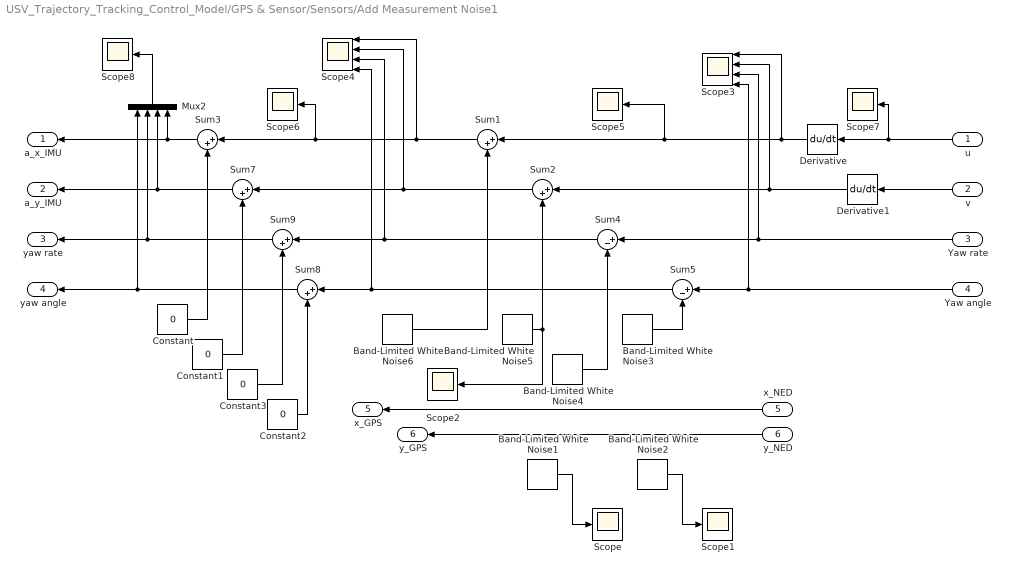
== system USV_Trajectory_Tracking_Control_Model/GPS & Sensor/Sensors/Add Measurement Noise1 ==
  u : Inport
  v : Inport  Port=2
  Yaw rate : Inport  Port=3
  Yaw angle : Inport  Port=4
  x_NED : Inport  Port=5
  y_NED : Inport  Port=6
  Band-Limited White Noise1 : simulink/Sources/Band-Limited White Noise  Cov=[0.5]  Ts=1  seed=[23341]
  Band-Limited White Noise2 : simulink/Sources/Band-Limited White Noise  Cov=[0.5]  Ts=1  seed=[23341]
  Band-Limited White Noise3 : simulink/Sources/Band-Limited White Noise  Cov=[0.0001]  Ts=0.1  seed=[23341]
  Band-Limited White Noise4 : simulink/Sources/Band-Limited White Noise  Cov=[0.00000001]  Ts=0.1  seed=[23341]
  Band-Limited White Noise5 : simulink/Sources/Band-Limited White Noise  Cov=[0.00000005]  Ts=0.1  seed=[23341]
  Band-Limited White Noise6 : simulink/Sources/Band-Limited White Noise  Cov=[0.000005]  Ts=0.1  seed=[23341]
  Constant{,1..3} (4 alike) : Constant  Value=0
  Derivative : Derivative
  Derivative1 : Derivative
  Mux2 : Mux
  Scope{,1..2,5..8} (7 alike) : Scope
  Scope3 : Scope  NumInputPorts=4
  Scope4 : Scope  NumInputPorts=4
  Sum{1..3,7..9} (6 alike) : Sum  Inputs=|++
  Sum4 : Sum  Inputs=|+-
  Sum5 : Sum  Inputs=|+-
  a_x_IMU : Outport  VectorParamsAs1DForOutWhenUnconnected=off
  a_y_IMU : Outport  Port=2  VectorParamsAs1DForOutWhenUnconnected=off
  yaw rate : Outport  Port=3  VectorParamsAs1DForOutWhenUnconnected=off
  yaw angle : Outport  Port=4  VectorParamsAs1DForOutWhenUnconnected=off
  x_GPS : Outport  Port=5  VectorParamsAs1DForOutWhenUnconnected=off
  y_GPS : Outport  Port=6  VectorParamsAs1DForOutWhenUnconnected=off
  wires:
  y_NED/1 -> y_GPS/1
  x_NED/1 -> x_GPS/1
  Band-Limited White Noise6/1 -> Sum1/2
  Sum2/1 -> Sum7/1, Scope4/2
  Sum4/1 -> Sum9/1, Scope4/3
  Band-Limited White Noise4/1 -> Sum4/2
  Sum5/1 -> Sum8/1, Scope4/4
  Band-Limited White Noise3/1 -> Sum5/2
  Sum1/1 -> Sum3/1, Scope6/1, Scope4/1
  Constant3/1 -> Sum9/2
  Sum9/1 -> yaw rate/1, Mux2/2
  Sum8/1 -> yaw angle/1, Mux2/1
  Yaw rate/1 -> Scope3/3, Sum4/1
  Sum7/1 -> a_y_IMU/1, Mux2/3
  Sum3/1 -> a_x_IMU/1, Mux2/4
  Mux2/1 -> Scope8/1
  Constant2/1 -> Sum8/2
  Constant1/1 -> Sum7/2
  Constant/1 -> Sum3/2
  Band-Limited White Noise2/1 -> Scope1/1
  Band-Limited White Noise1/1 -> Scope/1
  Derivative/1 -> Scope5/1, Sum1/1, Scope3/1
  Derivative1/1 -> Scope3/2, Sum2/1
  Yaw angle/1 -> Scope3/4, Sum5/1
  v/1 -> Derivative1/1
  u/1 -> Derivative/1, Scope7/1
  Band-Limited White Noise5/1 -> Sum2/2, Scope2/1

== system USV_Trajectory_Tracking_Control_Model/Tracking/Track error & Look ahead/Desire states ==
  x_desire : Inport
  y_desire : Inport  Port=2
  Derivative : Derivative
  Derivative1 : Derivative
  MATLAB Function : MATLAB Function  TreatAsAtomicUnit=on
  To Workspace : ToWorkspace  VariableName=x_desire  SampleTime=-1
  To Workspace1 : ToWorkspace  VariableName=y_desire  SampleTime=-1
  To Workspace2 : ToWorkspace  VariableName=yaw_desire  SampleTime=-1
  x_desire(t) : Outport  VectorParamsAs1DForOutWhenUnconnected=off
  y_desire(t) : Outport  Port=2  VectorParamsAs1DForOutWhenUnconnected=off
  yaw_desire(t) : Outport  Port=3  VectorParamsAs1DForOutWhenUnconnected=off
  wires:
  x_desire/1 -> Derivative/1, To Workspace/1, x_desire(t)/1
  y_desire/1 -> Derivative1/1, To Workspace1/1, y_desire(t)/1
  Derivative/1 -> MATLAB Function/1(dx)
  Derivative1/1 -> MATLAB Function/2(dy)
  MATLAB Function/1(yaw) -> To Workspace2/1, yaw_desire(t)/1

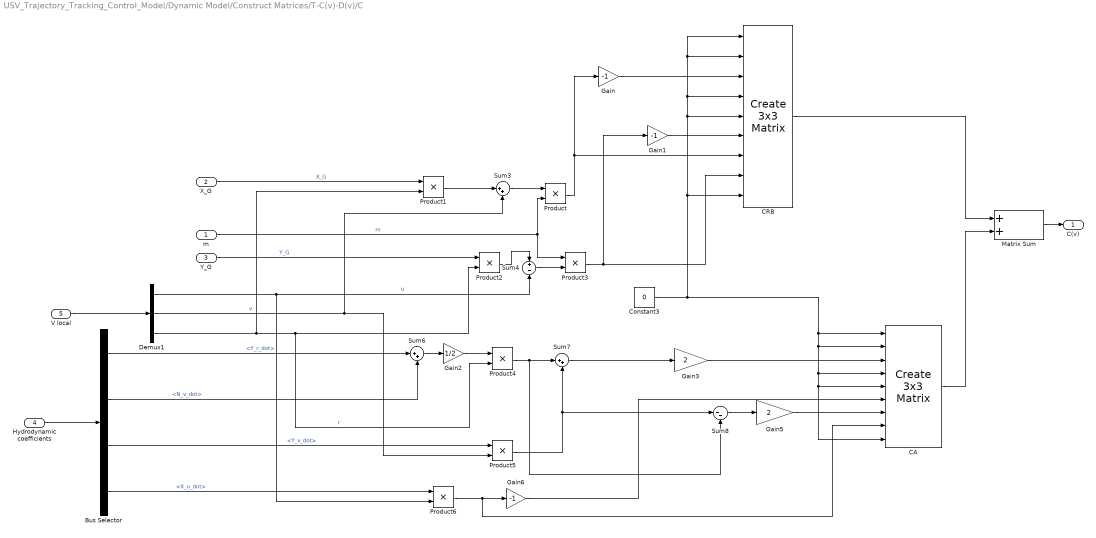
== system USV_Trajectory_Tracking_Control_Model/Dynamic Model/Construct Matrices/T-C(v)-D(v)/C ==
  m : Inport
  X_G : Inport  Port=2
  Y_G : Inport  Port=3
  Hydrodynamic coefficients : Inport  Port=4
  V local : Inport  Port=5
  " CRB" : sharedutil/Create 3x3 Matrix  aMode=aMode
      settings: SourceProductBaseCode=AE,PW,MT,UV,VE,VP
  Bus Selector : BusSelector  OutputSignals=Y_r_dot,N_v_dot,Y_v_dot,X_u_dot
  CA : sharedutil/Create 3x3 Matrix  aMode=aMode
      settings: SourceProductBaseCode=AE,PW,MT,UV,VE,VP
  Constant3 : Constant  Value=0
  Demux1 : Demux  Outputs=3
  Gain : Gain  Gain=-1
  Gain1 : Gain  Gain=-1
  Gain2 : Gain  Gain=1/2
  Gain3 : Gain  Gain=2
  Gain5 : Gain  Gain=2
  Gain6 : Gain  Gain=-1
  Matrix Sum : Sum
  Product{,1..6} (7 alike) : Product
  Sum3 : Sum  Inputs=|++
  Sum4 : Sum  Inputs=+-
  Sum6 : Sum  Inputs=|++
  Sum7 : Sum  Inputs=|++
  Sum8 : Sum  Inputs=|--
  C(v) : Outport  VectorParamsAs1DForOutWhenUnconnected=off
  wires:
  Bus Selector/1 -> Sum6/1  "<Y_r_dot>"
  Demux1/3 -> Product1/2, Product2/2, Product4/2  "r"
  Gain2/1 -> Product4/1
  CA/1 -> Matrix Sum/2
  Gain/1 -> " CRB"/3
  Bus Selector/2 -> Sum6/2  "<N_v_dot>"
  Sum3/1 -> Product/1
  Sum8/1 -> Gain5/1
  Product2/1 -> Sum4/1
  Sum6/1 -> Gain2/1
  Product5/1 -> Sum7/2, Sum8/1
  Gain1/1 -> " CRB"/6
  Product1/1 -> Sum3/1
  Y_G/1 -> Product2/1  "Y_G"
  Matrix Sum/1 -> C(v)/1
  Gain3/1 -> CA/3
  Gain6/1 -> CA/6
  Product6/1 -> Gain6/1, CA/8
  Demux1/2 -> Sum3/2, Product5/2  "v"
  Product4/1 -> Sum7/1, Sum8/2
  Product3/1 -> " CRB"/8, Gain1/1
  Gain5/1 -> CA/7
  " CRB"/1 -> Matrix Sum/1
  X_G/1 -> Product1/1  "X_G"
  Sum7/1 -> Gain3/1
  Product/1 -> " CRB"/7, Gain/1
  m/1 -> Product/2, Product3/1  "m"
  Constant3/1 -> " CRB"/5, " CRB"/4, " CRB"/2, " CRB"/1, " CRB"/9, CA/4, CA/5, CA/9, CA/2, CA/1
  Hydrodynamic coefficients/1 -> Bus Selector/1
  Bus Selector/4 -> Product6/1  "<X_u_dot>"
  Bus Selector/3 -> Product5/1  "<Y_v_dot>"
  Demux1/1 -> Sum4/2, Product6/2  "u"
  V local/1 -> Demux1/1
  Sum4/1 -> Product3/2

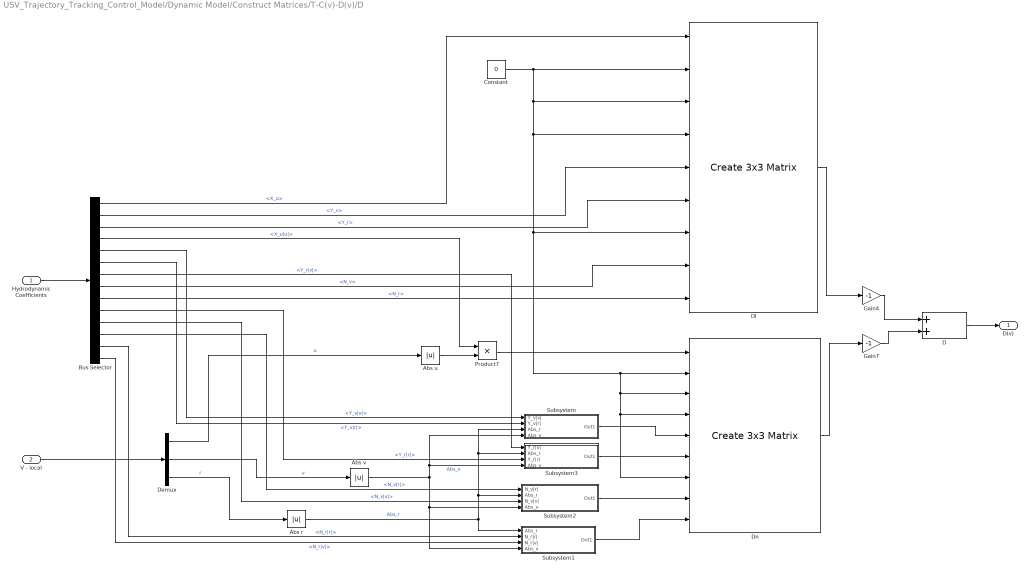
== system USV_Trajectory_Tracking_Control_Model/Dynamic Model/Construct Matrices/T-C(v)-D(v)/D ==
  Hydrodynamic Coefficients : Inport
  V - local : Inport  Port=2
  Abs r : Abs
  Abs u : Abs
  Abs v : Abs
  Bus Selector : BusSelector  OutputSignals=X_u,Y_v,Y_r,X_u|u|,Y_v|v|,Y_v|r|,Y_r|v|,N_v,N_r,Y_r|r|,N_v|v|,N_v|r|,N_r|r|,N_r|v|
  Constant : Constant  Value=0
  D : Sum
  Demux : Demux  Outputs=3
  Dl : sharedutil/Create 3x3 Matrix  aMode=aMode
      settings: SourceProductBaseCode=AE,PW,MT,UV,VE,VP
  Dn : sharedutil/Create 3x3 Matrix  aMode=aMode
      settings: SourceProductBaseCode=AE,PW,MT,UV,VE,VP
  Gain4 : Gain  Gain=-1
  Gain7 : Gain  Gain=-1
  Product7 : Product
  Subsystem : Subsystem
  Subsystem1 : Subsystem
  Subsystem2 : Subsystem
  Subsystem3 : Subsystem
  D(v) : Outport  VectorParamsAs1DForOutWhenUnconnected=off
  wires:
  Constant/1 -> Dn/7, Dn/4, Dn/3, Dn/2, Dl/7, Dl/4, Dl/3, Dl/2
  Abs u/1 -> Product7/2
  Abs r/1 -> Subsystem/3(Abs_r), Subsystem3/2("Abs_r "), Subsystem2/2(Abs_r), Subsystem1/1(Abs_r)  "Abs_r"
  Product7/1 -> Dn/1
  Abs v/1 -> Subsystem/4("Abs_v "), Subsystem3/4(Abs_v), Subsystem1/4(Abs_v), Subsystem2/4(Abs_v)  "Abs_v"
  Gain7/1 -> D/2
  Gain4/1 -> D/1
  Dl/1 -> Gain4/1
  Dn/1 -> Gain7/1
  D/1 -> D(v)/1
  Subsystem/1(Out1) -> Dn/5
  Subsystem1/1(Out1) -> Dn/9
  Subsystem2/1(Out1) -> Dn/8
  Subsystem3/1(Out1) -> Dn/6
  Hydrodynamic Coefficients/1 -> Bus Selector/1
  Bus Selector/5 -> Subsystem/1("Y_v|v| ")  "<Y_v|v|>"
  Bus Selector/6 -> Subsystem/2(Y_v|r|)  "<Y_v|r|>"
  Bus Selector/2 -> Dl/5  "<Y_v>"
  Bus Selector/7 -> Subsystem3/1(Y_r|v|)  "<Y_r|v|>"
  Bus Selector/10 -> Subsystem3/3(Y_r|r|)  "<Y_r|r|>"
  Bus Selector/11 -> Subsystem2/3(N_v|v|)  "<N_v|v|>"
  Bus Selector/8 -> Dl/8  "<N_v>"
  Bus Selector/12 -> Subsystem2/1(N_v|r|)  "<N_v|r|>"
  Bus Selector/14 -> Subsystem1/3(N_r|v|)  "<N_r|v|>"
  Bus Selector/9 -> Dl/9  "<N_r>"
  Bus Selector/13 -> Subsystem1/2(N_r|r|)  "<N_r|r|>"
  Bus Selector/1 -> Dl/1  "<X_u>"
  Bus Selector/4 -> Product7/1  "<X_u|u|>"
  Bus Selector/3 -> Dl/6  "<Y_r>"
  Demux/1 -> Abs u/1  "u"
  Demux/2 -> Abs v/1  "v"
  Demux/3 -> Abs r/1  "r"
  V - local/1 -> Demux/1

== system USV_Trajectory_Tracking_Control_Model/Dynamic Model/Construct Matrices/T-C(v)-D(v)/D/Subsystem ==
  "Y_v|v| " : Inport
  Y_v|r| : Inport  Port=2
  Abs_r : Inport  Port=3
  "Abs_v " : Inport  Port=4
  Product8 : Product
  Product9 : Product
  Sum10 : Sum  Inputs=|++
  Out1 : Outport  VectorParamsAs1DForOutWhenUnconnected=off
  wires:
  Y_v|r|/1 -> Product9/1
  Abs_r/1 -> Product9/2
  Product9/1 -> Sum10/2
  "Y_v|v| "/1 -> Product8/1
  Product8/1 -> Sum10/1
  "Abs_v "/1 -> Product8/2
  Sum10/1 -> Out1/1

== system USV_Trajectory_Tracking_Control_Model/Dynamic Model/Construct Matrices/T-C(v)-D(v)/D/Subsystem1 ==
  Abs_r : Inport
  N_r|r| : Inport  Port=2
  N_r|v| : Inport  Port=3
  Abs_v : Inport  Port=4
  Product14 : Product
  Product15 : Product
  Sum13 : Sum  Inputs=|++
  Out1 : Outport  VectorParamsAs1DForOutWhenUnconnected=off
  wires:
  Product15/1 -> Sum13/1
  Sum13/1 -> Out1/1
  N_r|v|/1 -> Product14/1
  Product14/1 -> Sum13/2
  Abs_r/1 -> Product15/2
  N_r|r|/1 -> Product15/1
  Abs_v/1 -> Product14/2

== system USV_Trajectory_Tracking_Control_Model/Dynamic Model/Construct Matrices/T-C(v)-D(v)/D/Subsystem2 ==
  N_v|r| : Inport
  Abs_r : Inport  Port=2
  N_v|v| : Inport  Port=3
  Abs_v : Inport  Port=4
  Product12 : Product
  Product13 : Product
  Sum12 : Sum  Inputs=|++
  Out1 : Outport  VectorParamsAs1DForOutWhenUnconnected=off
  wires:
  Sum12/1 -> Out1/1
  Product13/1 -> Sum12/1
  N_v|v|/1 -> Product12/1
  Product12/1 -> Sum12/2
  Abs_r/1 -> Product13/2
  Abs_v/1 -> Product12/2
  N_v|r|/1 -> Product13/1

== system USV_Trajectory_Tracking_Control_Model/Dynamic Model/Construct Matrices/T-C(v)-D(v)/D/Subsystem3 ==
  Y_r|v| : Inport
  "Abs_r " : Inport  Port=2
  Y_r|r| : Inport  Port=3
  Abs_v : Inport  Port=4
  Product10 : Product
  Product11 : Product
  Sum11 : Sum  Inputs=|++
  Out1 : Outport  VectorParamsAs1DForOutWhenUnconnected=off
  wires:
  Product11/1 -> Sum11/2
  Product10/1 -> Sum11/1
  Sum11/1 -> Out1/1
  Y_r|v|/1 -> Product10/1
  "Abs_r "/1 -> Product11/2
  Y_r|r|/1 -> Product11/1
  Abs_v/1 -> Product10/2

== matlab function USV_Trajectory_Tracking_Control_Model/Tracking/Track error & Look ahead/MATLAB Function3 ==
  data: k input; U_control output; U_d input; look_ahead input; along_e input; cross_e input
function U_control = fcn(k, U_d, look_ahead, along_e, cross_e)

U_control = (U_d+(k*along_e)) * ((cross_e^2 + look_ahead^2)^0.5) / look_ahead;

== matlab function USV_Trajectory_Tracking_Control_Model/RPM & PWM/PWM sim1 ==
  data: pwm_wave output double; rtime input; sig input
function pwm_wave   = fcn(rtime,sig)
%#PWM_generation
pwm_wave = 0;
saw = (rtime/.02 - floor(rtime/.02));
if sig<=saw
    pwm_wave=0;
elseif sig>saw
    pwm_wave=5;
end

== matlab function USV_Trajectory_Tracking_Control_Model/MATLAB Function ==
  data: x output; t input; y output
function [x,y] = fcn(t)

%Circle
x=50*sin(0.005*pi*t);
y=50*cos(0.005*pi*t)-50;


%Archimedean spiral
% x=0.1*t*sin(0.01*pi*t);
% y=0.1*t*cos(0.01*pi*t);

% Straight path
x=0.6*t;
y=0.7*t;

%Sine wave path
% x=0.1*pi*t;
% y=8*sin(0.1*x);

%parablol
% x=0.5*t;
% y=0.005*x^2;

== matlab function USV_Trajectory_Tracking_Control_Model/RPM & PWM/PWM sim2 ==
  data: pwm_wave output double; rtime input; sig input
function pwm_wave   = fcn(rtime,sig)
%#PWM_generation
pwm_wave = 0;
saw = (rtime/.02 - floor(rtime/.02));
if sig<=saw
    pwm_wave=0;
elseif sig>saw
    pwm_wave=5;
end

== matlab function USV_Trajectory_Tracking_Control_Model/Tracking/Target angle ==
  data: distance output; delta_x input; alpha output; delta_y input
function [distance,alpha] = fcn(delta_x, delta_y)

alpha = atan2(delta_y,delta_x);
distance = ((delta_x^2)+(delta_y^2))^0.5;

== matlab function USV_Trajectory_Tracking_Control_Model/GPS & Sensor/Frame Transformation/MATLAB Function ==
  data: u input; Vx_0 output; v input; Yaw input; Vy_0 output
function [Vx_0 , Vy_0 ] = fcn(u, v, Yaw)

Vx_0 =  cos(Yaw)*u - sin(Yaw)*v ;
Vy_0 =  sin(Yaw)*u + cos(Yaw)*v ;

== matlab function USV_Trajectory_Tracking_Control_Model/Tracking/MATLAB Function ==
  data: alpha input; delta output; psi input
function delta = fcn(alpha, psi)

delta_1 = alpha - psi;
delta = delta_1;
delta_2 = delta_1 - 2*pi;

if (delta_1<0)
    delta_2 = delta_1 - 2*pi;
end

if abs(delta)>pi
    delta = delta_2;
end

== matlab function USV_Trajectory_Tracking_Control_Model/Tracking/Surge Velocity Control ==
  data: U_control input; u_Control output; u_low input; approach input; high_speed input; maneuver input
function u_Control  = fcn(U_control, u_low,approach,high_speed,maneuver)

u_Control = (u_low*maneuver + high_speed* U_control)*approach;

== matlab function USV_Trajectory_Tracking_Control_Model/Tracking/Track error & Look ahead/Desire states/MATLAB Function ==
  data: dx input; yaw output; dy input
function yaw = fcn(dx,dy)

yaw = atan2(dy,dx);

== matlab function USV_Trajectory_Tracking_Control_Model/Tracking/Track error & Look ahead/MATLAB Function ==
  data: look_ahead input; x_target output; x_desire input; y_desire input; yaw input; y_target output
function [x_target, y_target] = fcn(look_ahead, x_desire, y_desire, yaw)

x_target = x_desire + (look_ahead*cos(yaw));
y_target = y_desire + (look_ahead*sin(yaw));

== matlab function USV_Trajectory_Tracking_Control_Model/Tracking/Track error & Look ahead/MATLAB Function1 ==
  data: yaw input; along_e output; delta_x input; delta_y input; cross_e output
function [along_e, cross_e] = fcn(yaw, delta_x, delta_y)

along_e = (cos(yaw)*delta_x) + (sin(yaw)*delta_y);
cross_e = (-sin(yaw)*delta_x) + (cos(yaw)*delta_y);

== matlab function USV_Trajectory_Tracking_Control_Model/Tracking/Track error & Look ahead/MATLAB Function2 ==
  data: Vx_d input; U_d output; Vy_d input
function U_d = fcn(Vx_d, Vy_d)

U_d = ((Vx_d^2) + (Vy_d^2))^0.5;
